simulink model "mc64_hb_43_newquant"  (Simulink 7.6)
settings: Solver=ode45  StartTime=0.0  StopTime=5000  RelTol=1e-3
libraries: xbsIndex_r4 x1281, xps_library x27, casper_library_misc x17, dspsigops x8
(part 2 of 13)

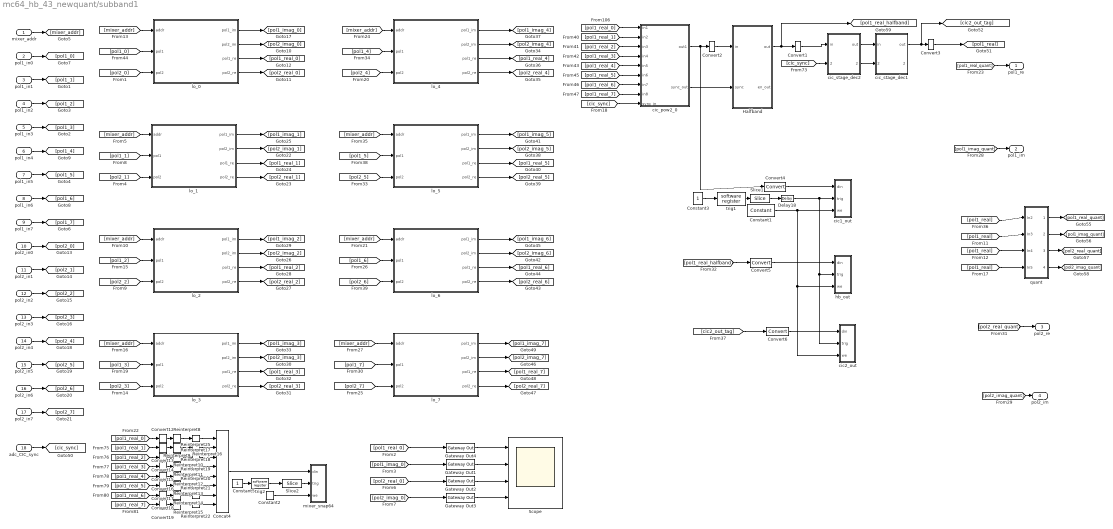
== system mc64_hb_43_newquant/subband1 ==
  mixer_addr : Inport
  pol1_in0 : Inport  Port=2
  pol1_in1 : Inport  Port=3
  pol1_in2 : Inport  Port=4
  pol1_in3 : Inport  Port=5
  pol1_in4 : Inport  Port=6
  pol1_in5 : Inport  Port=7
  pol1_in6 : Inport  Port=8
  pol1_in7 : Inport  Port=9
  pol2_in0 : Inport  Port=10
  pol2_in1 : Inport  Port=11
  pol2_in2 : Inport  Port=12
  pol2_in3 : Inport  Port=13
  pol2_in4 : Inport  Port=14
  pol2_in5 : Inport  Port=15
  pol2_in6 : Inport  Port=16
  pol2_in7 : Inport  Port=17
  adc_CIC_sync : Inport  Port=18
  Concat4 : xbsIndex_r4/Concat  num_inputs=8  dbl_ovrd=off  block_type=concat
  Constant1 : xbsIndex_r4/Constant  const=1  gui_display_data_type=Boolean  arith_type=Boolean  n_bits=16  bin_pt=14  preci_type=Single  exp_width=8  frac_width=24  explicit_period=off  period=1  equ=P=C  opselect=C  inp2=PCIN>>17  opr=+  inp1=P  carry=CIN  dbl_ovrd=off  block_type=constant
  Constant2 : xbsIndex_r4/Constant  const=1  gui_display_data_type=Boolean  arith_type=Boolean  n_bits=16  bin_pt=14  preci_type=Single  exp_width=8  frac_width=24  explicit_period=off  period=1  equ=P=C  opselect=C  inp2=PCIN>>17  opr=+  inp1=P  carry=CIN  dbl_ovrd=off  block_type=constant
  Constant3 : Constant
  Constant5 : Constant
  Convert1 : xbsIndex_r4/Convert  gui_display_data_type=Fixed-point  arith_type="Signed  (2's comp)"  n_bits=32  bin_pt=12  float_type=Single  exp_bits=8  fraction_bits=24  quantization=Truncate  overflow=Wrap  en=off  latency=1  dbl_ovrd=off  pipeline=off  block_type=convert
  Convert{12..19} (8 alike) : xbsIndex_r4/Convert  gui_display_data_type=Fixed-point  arith_type=Unsigned  n_bits=8  bin_pt=6  float_type=Single  exp_bits=8  fraction_bits=24  quantization=Truncate  overflow=Wrap  en=off  latency=2  dbl_ovrd=off  pipeline=off  block_type=convert
      settings: block_version=11.4
  Convert2 : xbsIndex_r4/Convert  gui_display_data_type=Fixed-point  arith_type="Signed  (2's comp)"  n_bits=32  bin_pt=18  float_type=Single  exp_bits=8  fraction_bits=24  quantization=Truncate  overflow=Wrap  en=off  latency=1  dbl_ovrd=off  pipeline=off  block_type=convert
  Convert3 : xbsIndex_r4/Convert  gui_display_data_type=Fixed-point  arith_type="Signed  (2's comp)"  n_bits=32  bin_pt=6  float_type=Single  exp_bits=8  fraction_bits=24  quantization=Truncate  overflow=Wrap  en=off  latency=1  dbl_ovrd=off  pipeline=off  block_type=convert
  Convert4 : xbsIndex_r4/Convert  gui_display_data_type=Fixed-point  arith_type="Signed  (2's comp)"  n_bits=64  bin_pt=22  float_type=Single  exp_bits=8  fraction_bits=24  quantization=Truncate  overflow=Wrap  en=off  latency=1  dbl_ovrd=off  pipeline=off  block_type=convert
  Convert5 : xbsIndex_r4/Convert  gui_display_data_type=Fixed-point  arith_type="Signed  (2's comp)"  n_bits=64  bin_pt=32  float_type=Single  exp_bits=8  fraction_bits=24  quantization=Truncate  overflow=Wrap  en=off  latency=1  dbl_ovrd=off  pipeline=off  block_type=convert
  Convert6 : xbsIndex_r4/Convert  gui_display_data_type=Fixed-point  arith_type="Signed  (2's comp)"  n_bits=64  bin_pt=12  float_type=Single  exp_bits=8  fraction_bits=24  quantization=Truncate  overflow=Wrap  en=off  latency=1  dbl_ovrd=off  pipeline=off  block_type=convert
  Delay18 : xbsIndex_r4/Delay  rst=off  infoeditControl=Selection of Reset will increase slice count due to use of real FFs and instead of SRLs  en=off  latency=20  dbl_ovrd=off  reg_retiming=off  block_type=delay
  Gateway Out{1..4} (4 alike) : xbsIndex_r4/Gateway Out  hdl_port=on  timing_constraint=None  locs_specified=off  LOCs={}  block_type=gatewayout
      settings: infoedit="Gateway out block.  Converts Xilinx fixed point or floating-point type inputs into ouputs of type Simulink integer, double, or fixed point.<br><br>Hardware notes:  In hardware these blocks become top level output ports or are discarded, depending on how they are configured."
  Halfband : Subsystem  AncestorBlock=gbt_library/Halfband  mask(Halfband FIR){mult_latency=3, add_latency=2, hold_period=2, passband=0.4, fir_len=17}
      mask prompts: mult_latency "Multiplication latency"; add_latency "Add latency"; hold_period "Hold Period"; passband "Width of Halfband passband (<0.5)"; fir_len "FIR Length (odd) [Number of Taps will be: 2*fir_len+1]"
      mask help: A halfband FIR for low rate computation.
      mask init:
      | coeffs = halfband_coeff_gen(fir_len, passband);
      | config.source=str2func('hold_fir_init_xblock');
      | config.depend=[get_dependlist('hold_fir'),{'halfband_coeff_gen'}];
      | config.toplevel=gcb;
      | set_param(gcb,'LinkStatus','inactive');
      | xBlock(config, {config.toplevel,...
      |     'mult_latency', mult_latency, ...
      |     'add_latency', add_latency, ...
      |     'hold_period', hold_period, ...
      |     'coeffs', coeffs});
      settings: AttributesFormatString=|
      | 35-tap FIR filter (19 nonzero tap)
      |  hold period: 2
      |  mult latency: 3
      |  add latency: 2
  Reinterpret{8..15} (8 alike) : xbsIndex_r4/Reinterpret  force_arith_type=on  arith_type="Signed  (2's comp)"  force_bin_pt=on  bin_pt=7  block_type=reinterpret
  Reinterpret{16..22,25} (8 alike) : xbsIndex_r4/Reinterpret  force_arith_type=on  arith_type=Unsigned  force_bin_pt=on  bin_pt=0  block_type=reinterpret
  Scope : Scope  NumInputPorts=4
      settings: YMin=-0.0075~-1~-0.0075~-1  YMax=0.0075~1~0.0075~1
  Slice1 : xbsIndex_r4/Slice  nbits=1  boolean_output=on  mode=Lower Bit Location + Width  bit1=0  base1=MSB of Input  bit0=0  base0=LSB of Input  dbl_ovrd=off  block_type=slice
  Slice2 : xbsIndex_r4/Slice  nbits=1  boolean_output=on  mode=Lower Bit Location + Width  bit1=0  base1=MSB of Input  bit0=0  base0=LSB of Input  dbl_ovrd=off  block_type=slice
  cic1_out : Subsystem  AncestorBlock=casper_library_scopes/snap64  mask(snap64){nsamples=13}
      mask prompts: nsamples "No. of samples(2^?)"
      mask help:
      | The <i>snap</i> block provides a packaged solution to capturing data from
      | the FPGA fabric and making it accessible from the CPU.  The block comes in
      | 2 flavors: <i>snap</i> (which captures to a 32 bit wide Shared BRAM), and
      | <i>snap64</i> (which captures to 2x32 bit wide Shared BRAMs to effect a
      | 64 bit capture).
      mask Help: eval('xlWeb(''http://casper.berkeley.edu/wiki/Snap'')')
  cic2_out : Subsystem  AncestorBlock=casper_library_scopes/snap64  mask(snap64){nsamples=13}
      mask prompts: nsamples "No. of samples(2^?)"
      mask help:
      | The <i>snap</i> block provides a packaged solution to capturing data from
      | the FPGA fabric and making it accessible from the CPU.  The block comes in
      | 2 flavors: <i>snap</i> (which captures to a 32 bit wide Shared BRAM), and
      | <i>snap64</i> (which captures to 2x32 bit wide Shared BRAMs to effect a
      | 64 bit capture).
      mask Help: eval('xlWeb(''http://casper.berkeley.edu/wiki/Snap'')')
  cic_pow2_0 : Subsystem  AncestorBlock=gbt_library/cic_pow2  mask(CIC (pow2)){n_stages=4, dec_rate=16, input_clk_period=1, n_inputs=8, add_latency=1, n_bits=8, bin_pt=7}
      mask prompts: n_stages "CIC filter Order"; dec_rate "Decimation rate"; input_clk_period "Input Clock Period"; n_inputs "Number of inputs"; add_latency "Add latency"; n_bits "Input bit width"; bin_pt "Binary point"
      mask help:
      | A non-recursive CIC filter with parallel inputs.
      | Supports decimation rate of power of 2.
      | A multi-stage implementation with each stage of decimation rate 2.
      mask init:
      | config.source = str2func('cic_pow2_init_xblock');
      | config.toplevel = gcb;
      | config.depend = get_dependlist('cic_pow2'); 
      | set_param(gcb,'LinkStatus','inactive');
      | xBlock(config, {config.toplevel,...
      |                 'n_stages',n_stages, ...
      |                 'dec_rate', dec_rate, ...
      |                 'input_clk_rate', input_clk_period, ...
      |                 'n_inputs', n_inputs,...
      |                 'add_latency',add_latency,...
      |                 'n_bits', n_bits, ...
      |                 'bin_pt', bin_pt} ...
      |                 );
      | disp('new block added');
      settings: AttributesFormatString=|
      | dec_rate = 16
      | Order = 4
  cic_stage_dec1 : Subsystem  AncestorBlock=gbt_library/cic_stage_dec2  mask(CIC stage (dec2)){n_stages=3, recursive=off, dec_rate=2, n_inputs=1, input_clk_period=1, input_period=4, add_latency=2, n_bits=8, bin_pt=7}
      mask prompts: n_stages "CIC filter Order"; recursive "Recursive?"; dec_rate "Decimation rate"; n_inputs "Number of Inputs"; input_clk_period "Input Clock period (Actual)"; input_period "Effective Input Sampling Period"; add_latency "Add latency"; n_bits "Input bit width"; bin_pt "Binary point"
      mask help:
      | A single stage of CIC filter with even number of parallel inputs.
      | Only supports decimation rate = 2.
      | If n_inputs > 1, number of outputs = n_inputs/2.
      | Non-recursive.
      |
      | Clock period:
      | input_clk_period is the actual sampling period of incoming data stream.
      | input_period is the effective (or expected) sampling period of incoming data stream.
      | E.g. For incoming data stream X[n] = [1& 1 2 2 3 3 4 4 5 5 ...], the input_clk_period is 1 and the input_period is 2.
      mask init:
      | if recursive
      |     % recursive case
      |     config.source=str2func('cic_stage_dec2_recursive_init_xblock');
      |     config.toplevel=gcb;
      |     config.depend = get_dependlist('cic_stage_dec2_recursive');
      |     set_param(gcb,'LinkStatus','inactive');
      |     xBlock(config, {config.toplevel, ...
      |                 'n_stages', n_stages, ...
      |                 'dec_rate', dec_rate, ...
      |                 'n_inputs', n_inputs, ...
      |                 'input_clk_period', input_clk_period, ...
      |                 'input_period', input_period, ...
      |                 'add_latency', add_latency, ...
      |                 'input_bits', n_bits, ...
      |                 'bin_pt', bin_pt, ...
      |                 'delay_len', 1});
      | else
      |     % non-recursive case
      |     config.source=str2func('cic_stage_dec2_init_xblock');
      |     config.toplevel=gcb;
      |     config.depend = get_dependlist('cic_stage_dec2');
      |     set_param(gcb,'LinkStatus','inactive');
      |     xBlock(config, {config.toplevel, ...
      |                 'n_stages', n_stages, ...
      |                 'dec_rate', dec_rate, ...
      |                 'n_inputs', n_inputs, ...
      |                 'input_clk_period', input_clk_period, ...
      |                 'input_period', input_period, ...
      |                 'add_latency', add_latency, ...
      |                 'n_bits', n_bits, ...
      |                 'bin_pt', bin_pt});
      | end
      settings: AttributesFormatString=|
      | nonrecursive
      | 8_7_in
      | clock(actualy/effective): 1/4
      mask CallbackString:
      | ||n=get_param(gcb,'dec_rate');
      | if ~isempty(n)
      |     n = eval(n);
      |     if ~isprime(n) && n~=1
      |         errordlg('Only supports decimation rate that is a prime number or 1');
      |         set_param(gcb,'dec_rate','');
      |     end
      | end||||||
  cic_stage_dec2 : Subsystem  AncestorBlock=gbt_library/cic_stage_dec2  mask(CIC stage (dec2)){n_stages=3, recursive=off, dec_rate=2, n_inputs=1, input_clk_period=1, input_period=2, add_latency=2, n_bits=8, bin_pt=7}
      mask prompts: n_stages "CIC filter Order"; recursive "Recursive?"; dec_rate "Decimation rate"; n_inputs "Number of Inputs"; input_clk_period "Input Clock period (Actual)"; input_period "Effective Input Sampling Period"; add_latency "Add latency"; n_bits "Input bit width"; bin_pt "Binary point"
      mask help:
      | A single stage of CIC filter with even number of parallel inputs.
      | Only supports decimation rate = 2.
      | If n_inputs > 1, number of outputs = n_inputs/2.
      | Non-recursive.
      |
      | Clock period:
      | input_clk_period is the actual sampling period of incoming data stream.
      | input_period is the effective (or expected) sampling period of incoming data stream.
      | E.g. For incoming data stream X[n] = [1& 1 2 2 3 3 4 4 5 5 ...], the input_clk_period is 1 and the input_period is 2.
      mask init: same as mc64_hb_43_newquant/subband1/cic_stage_dec1
      settings: AttributesFormatString=|
      | nonrecursive
      | 8_7_in
      | clock(actualy/effective): 1/2
      mask CallbackString:
      | ||n=get_param(gcb,'dec_rate');
      | if ~isempty(n)
      |     n = eval(n);
      |     if ~isprime(n) && n~=1
      |         errordlg('Only supports decimation rate that is a prime number or 1');
      |         set_param(gcb,'dec_rate','');
      |     end
      | end||||||
  hb_out : Subsystem  AncestorBlock=casper_library_scopes/snap64  mask(snap64){nsamples=13}
      mask prompts: nsamples "No. of samples(2^?)"
      mask help:
      | The <i>snap</i> block provides a packaged solution to capturing data from
      | the FPGA fabric and making it accessible from the CPU.  The block comes in
      | 2 flavors: <i>snap</i> (which captures to a 32 bit wide Shared BRAM), and
      | <i>snap64</i> (which captures to 2x32 bit wide Shared BRAMs to effect a
      | 64 bit capture).
      mask Help: eval('xlWeb(''http://casper.berkeley.edu/wiki/Snap'')')
  lo_0 : Subsystem  AncestorBlock=gbt_library/complex_mix_lo
  lo_1 : Subsystem  AncestorBlock=gbt_library/complex_mix_lo
  lo_2 : Subsystem  AncestorBlock=gbt_library/complex_mix_lo
  lo_3 : Subsystem  AncestorBlock=gbt_library/complex_mix_lo
  lo_4 : Subsystem  AncestorBlock=gbt_library/complex_mix_lo
  lo_5 : Subsystem  AncestorBlock=gbt_library/complex_mix_lo
  lo_6 : Subsystem  AncestorBlock=gbt_library/complex_mix_lo
  lo_7 : Subsystem  AncestorBlock=gbt_library/complex_mix_lo
  mixer_snap64 : Subsystem  AncestorBlock=casper_library_scopes/snap64  mask(snap64){nsamples=11}
      mask prompts: nsamples "No. of samples(2^?)"
      mask help:
      | The <i>snap</i> block provides a packaged solution to capturing data from
      | the FPGA fabric and making it accessible from the CPU.  The block comes in
      | 2 flavors: <i>snap</i> (which captures to a 32 bit wide Shared BRAM), and
      | <i>snap64</i> (which captures to 2x32 bit wide Shared BRAMs to effect a
      | 64 bit capture).
      mask Help: eval('xlWeb(''http://casper.berkeley.edu/wiki/Snap'')')
  quant : Subsystem
  trig1 : xps_library/software register  Tag=xps:sw_reg  SystemSampleTime=-1  io_dir=From Processor  arith_type=Unsigned  bitwidth=32  bin_pt=0  sample_period=1  gw_name=mc64_hb_43_noise_subband1_trig1_user_data_out
      link override cic_filter_testing_to_compile_trig_user_data_out: arith_type=Unsigned  n_bits=32  bin_pt=0  period=1
  trig2 : xps_library/software register  Tag=xps:sw_reg  SystemSampleTime=-1  io_dir=From Processor  arith_type=Unsigned  bitwidth=32  bin_pt=0  sample_period=1  gw_name=mc64_hb_43_noise_subband1_trig2_user_data_out
      link override cic_filter_testing_to_compile_trig_user_data_out: arith_type=Unsigned  n_bits=32  bin_pt=0  period=1
  pol1_re : Outport
  pol1_im : Outport  Port=2
  pol2_re : Outport  Port=3
  pol2_im : Outport  Port=4
  wires:
  mixer_addr/1 -> [mixer_addr]
  pol1_in0/1 -> [pol1_0]
  [pol1_real_0] -> cic_pow2_0/1(in1)
  pol1_in1/1 -> [pol1_1]
  pol1_in2/1 -> [pol1_2]
  pol1_in3/1 -> [pol1_3]
  pol1_in4/1 -> [pol1_4]
  pol1_in5/1 -> [pol1_5]
  pol1_in6/1 -> [pol1_6]
  pol1_in7/1 -> [pol1_7]
  pol2_in0/1 -> [pol2_0]
  pol2_in1/1 -> [pol2_1]
  pol2_in2/1 -> [pol2_2]
  pol2_in3/1 -> [pol2_3]
  pol2_in4/1 -> [pol2_4]
  pol2_in5/1 -> [pol2_5]
  pol2_in6/1 -> [pol2_6]
  pol2_in7/1 -> [pol2_7]
  [mixer_addr] -> lo_1/1(addr)
  [mixer_addr] -> lo_2/1(addr)
  [mixer_addr] -> lo_3/1(addr)
  [pol1_real_1] -> cic_pow2_0/2(in2)
  [pol1_real_2] -> cic_pow2_0/3(in3)
  [pol1_real_3] -> cic_pow2_0/4(in4)
  [pol1_real_4] -> cic_pow2_0/5(in5)
  [pol1_real_5] -> cic_pow2_0/6(in6)
  [pol1_real_6] -> cic_pow2_0/7(in7)
  [pol1_real_7] -> cic_pow2_0/8(in8)
  lo_4/1(pol1_im) -> [pol1_imag_4]
  lo_4/2(pol2_im) -> [pol2_imag_4]
  lo_4/3(pol1_re) -> [pol1_real_4]
  lo_4/4(pol2_re) -> [pol2_real_4]
  [mixer_addr] -> lo_4/1(addr)
  [pol2_4] -> lo_4/3(pol2)
  [pol1_4] -> lo_4/2(pol1)
  [mixer_addr] -> lo_0/1(addr)
  [pol1_0] -> lo_0/2(pol1)
  [pol2_0] -> lo_0/3(pol2)
  lo_0/1(pol1_im) -> [pol1_imag_0]
  lo_0/2(pol2_im) -> [pol2_imag_0]
  lo_0/3(pol1_re) -> [pol1_real_0]
  lo_0/4(pol2_re) -> [pol2_real_0]
  [pol1_1] -> lo_1/2(pol1)
  [pol2_1] -> lo_1/3(pol2)
  lo_1/1(pol1_im) -> [pol1_imag_1]
  lo_1/2(pol2_im) -> [pol2_imag_1]
  lo_1/3(pol1_re) -> [pol1_real_1]
  lo_1/4(pol2_re) -> [pol2_real_1]
  [pol1_2] -> lo_2/2(pol1)
  [pol2_2] -> lo_2/3(pol2)
  [pol1_3] -> lo_3/2(pol1)
  [pol2_3] -> lo_3/3(pol2)
  lo_3/1(pol1_im) -> [pol1_imag_3]
  lo_3/2(pol2_im) -> [pol2_imag_3]
  lo_3/3(pol1_re) -> [pol1_real_3]
  lo_3/4(pol2_re) -> [pol2_real_3]
  [mixer_addr] -> lo_5/1(addr)
  [pol1_5] -> lo_5/2(pol1)
  [pol2_5] -> lo_5/3(pol2)
  lo_5/1(pol1_im) -> [pol1_imag_5]
  lo_5/2(pol2_im) -> [pol2_imag_5]
  lo_5/3(pol1_re) -> [pol1_real_5]
  lo_5/4(pol2_re) -> [pol2_real_5]
  [mixer_addr] -> lo_6/1(addr)
  [pol1_6] -> lo_6/2(pol1)
  [pol2_6] -> lo_6/3(pol2)
  lo_6/1(pol1_im) -> [pol1_imag_6]
  lo_6/2(pol2_im) -> [pol2_imag_6]
  lo_6/3(pol1_re) -> [pol1_real_6]
  lo_6/4(pol2_re) -> [pol2_real_6]
  [mixer_addr] -> lo_7/1(addr)
  [pol1_7] -> lo_7/2(pol1)
  [pol2_7] -> lo_7/3(pol2)
  lo_7/1(pol1_im) -> [pol1_imag_7]
  lo_7/2(pol2_im) -> [pol2_imag_7]
  lo_7/3(pol1_re) -> [pol1_real_7]
  lo_7/4(pol2_re) -> [pol2_real_7]
  lo_2/1(pol1_im) -> [pol1_imag_2]
  lo_2/2(pol2_im) -> [pol2_imag_2]
  lo_2/3(pol1_re) -> [pol1_real_2]
  lo_2/4(pol2_re) -> [pol2_real_2]
  [pol1_real_0] -> Gateway Out4/1
  [pol1_imag_0] -> Gateway Out1/1
  [pol2_real_0] -> Gateway Out2/1
  [pol2_imag_0] -> Gateway Out3/1
  Gateway Out4/1 -> Scope/1
  Gateway Out1/1 -> Scope/2
  Gateway Out2/1 -> Scope/3
  Gateway Out3/1 -> Scope/4
  adc_CIC_sync/1 -> [cic_sync]
  [cic_sync] -> cic_pow2_0/9(sync_in)
  Concat4/1 -> mixer_snap64/1(din)
  Constant2/1 -> mixer_snap64/3(we)
  Convert12/1 -> Reinterpret8/1
  [pol1_real_0] -> Convert12/1
  Reinterpret8/1 -> Reinterpret25/1
  Convert13/1 -> Reinterpret9/1
  [pol1_real_1] -> Convert13/1
  Reinterpret9/1 -> Reinterpret16/1
  Convert14/1 -> Reinterpret10/1
  [pol1_real_2] -> Convert14/1
  Reinterpret10/1 -> Reinterpret17/1
  Convert15/1 -> Reinterpret11/1
  [pol1_real_3] -> Convert15/1
  Reinterpret11/1 -> Reinterpret18/1
  Convert16/1 -> Reinterpret12/1
  [pol1_real_4] -> Convert16/1
  Reinterpret12/1 -> Reinterpret19/1
  Convert17/1 -> Reinterpret13/1
  [pol1_real_5] -> Convert17/1
  Reinterpret13/1 -> Reinterpret20/1
  Convert18/1 -> Reinterpret14/1
  [pol1_real_6] -> Convert18/1
  Reinterpret14/1 -> Reinterpret21/1
  Convert19/1 -> Reinterpret15/1
  [pol1_real_7] -> Convert19/1
  Reinterpret15/1 -> Reinterpret22/1
  Reinterpret25/1 -> Concat4/1
  Reinterpret16/1 -> Concat4/2
  Reinterpret17/1 -> Concat4/3
  Reinterpret18/1 -> Concat4/4
  Reinterpret19/1 -> Concat4/5
  Reinterpret20/1 -> Concat4/6
  Reinterpret21/1 -> Concat4/7
  Reinterpret22/1 -> Concat4/8
  Constant5/1 -> trig2/1
  trig2/1 -> Slice2/1
  Slice2/1 -> mixer_snap64/2(trig)
  [pol1_real_quant] -> pol1_re/1
  cic_pow2_0/2(sync_out) -> Halfband/2(sync)
  cic_stage_dec2/2(sync_out) -> cic_stage_dec1/2(sync_in)
  cic_stage_dec2/1(out) -> cic_stage_dec1/1(in)
  Halfband/1(out) -> Convert1/1, [pol1_real_halfband]
  cic_stage_dec1/1(out) -> Convert3/1, [cic2_out_tag]
  [cic_sync] -> cic_stage_dec2/2(sync_in)
  cic_pow2_0/1(out1) -> Convert2/1, Convert4/1
  Convert2/1 -> Halfband/1(in)
  Convert1/1 -> cic_stage_dec2/1(in)
  Convert3/1 -> [pol1_real]
  [pol1_imag_quant] -> pol1_im/1
  quant/1(Out1) -> [pol1_real_quant]
  quant/2(Out2) -> [pol1_imag_quant]
  [pol1_real] -> quant/1(In2)
  [pol1_real] -> quant/2(In3)
  [pol1_real] -> quant/3(In4)
  [pol1_real] -> quant/4(In5)
  quant/3(Out3) -> [pol2_real_quant]
  quant/4(Out4) -> [pol2_imag_quant]
  [pol2_real_quant] -> pol2_re/1
  [pol2_imag_quant] -> pol2_im/1
  Constant1/1 -> cic1_out/3(we), hb_out/3(we), cic2_out/3(we)
  Constant3/1 -> trig1/1
  trig1/1 -> Slice1/1
  Slice1/1 -> Delay18/1
  Delay18/1 -> cic1_out/2(trig), hb_out/2(trig), cic2_out/2(trig)
  Convert4/1 -> cic1_out/1(din)
  [pol1_real_halfband] -> Convert5/1
  Convert5/1 -> hb_out/1(din)
  [cic2_out_tag] -> Convert6/1
  Convert6/1 -> cic2_out/1(din)

== system mc64_hb_43_newquant/adc083000x2/adc0_sim ==
  sim_adc_data_in : Inport
  adc_bias : Bias  Bias=128  SaturateOnIntegerOverflow=on
  adc_gain : Gain  Gain=128
  overflow_detector : Subsystem  AncestorBlock=casper_library/Misc/of_detect_bus  mask(of_detect_bus){nStreams=8, bit_width=8}
      mask prompts: nStreams "Number of Streams"; bit_width "Bit Width"
      mask init:
      | adc_overflow_detector_init(gcb, ...
      |     'nStreams', nStreams, ...
      |     'bit_width', bit_width);
  sample0_ds : dspsigops/Downsample  N=8  phase=1  InputProcessing=Inherited (this choice will be removed - see release notes)  RateOptions=Enforce single-rate processing  smode=Force single rate  fmode=Maintain input frame size  ic=0
  sample1_ds : dspsigops/Downsample  N=8  phase=2  InputProcessing=Inherited (this choice will be removed - see release notes)  RateOptions=Enforce single-rate processing  smode=Force single rate  fmode=Maintain input frame size  ic=0
  sample2_ds : dspsigops/Downsample  N=8  phase=3  InputProcessing=Inherited (this choice will be removed - see release notes)  RateOptions=Enforce single-rate processing  smode=Force single rate  fmode=Maintain input frame size  ic=0
  sample3_ds : dspsigops/Downsample  N=8  phase=4  InputProcessing=Inherited (this choice will be removed - see release notes)  RateOptions=Enforce single-rate processing  smode=Force single rate  fmode=Maintain input frame size  ic=0
  sample4_ds : dspsigops/Downsample  N=8  phase=5  InputProcessing=Inherited (this choice will be removed - see release notes)  RateOptions=Enforce single-rate processing  smode=Force single rate  fmode=Maintain input frame size  ic=0
  sample5_ds : dspsigops/Downsample  N=8  phase=6  InputProcessing=Inherited (this choice will be removed - see release notes)  RateOptions=Enforce single-rate processing  smode=Force single rate  fmode=Maintain input frame size  ic=0
  sample6_ds : dspsigops/Downsample  N=8  phase=7  InputProcessing=Inherited (this choice will be removed - see release notes)  RateOptions=Enforce single-rate processing  smode=Force single rate  fmode=Maintain input frame size  ic=0
  sample7_ds : dspsigops/Downsample  N=8  phase=0  InputProcessing=Inherited (this choice will be removed - see release notes)  RateOptions=Enforce single-rate processing  smode=Force single rate  fmode=Maintain input frame size  ic=0
  s0 : Outport
  s1 : Outport  Port=2
  s2 : Outport  Port=3
  s3 : Outport  Port=4
  s4 : Outport  Port=5
  s5 : Outport  Port=6
  s6 : Outport  Port=7
  s7 : Outport  Port=8
  of : Outport  Port=9
  wires:
  sim_adc_data_in/1 -> adc_gain/1
  adc_gain/1 -> adc_bias/1
  overflow_detector/1(overflow) -> of/1
  adc_bias/1 -> sample0_ds/1, sample1_ds/1, sample2_ds/1, sample3_ds/1, sample4_ds/1, sample5_ds/1, sample6_ds/1, sample7_ds/1
  sample0_ds/1 -> overflow_detector/1(s0), s0/1
  sample1_ds/1 -> overflow_detector/2(s1), s1/1
  sample2_ds/1 -> overflow_detector/3(s2), s2/1
  sample3_ds/1 -> overflow_detector/4(s3), s3/1
  sample4_ds/1 -> overflow_detector/5(s4), s4/1
  sample5_ds/1 -> overflow_detector/6(s5), s5/1
  sample6_ds/1 -> overflow_detector/7(s6), s6/1
  sample7_ds/1 -> overflow_detector/8(s7), s7/1

== system mc64_hb_43_newquant/adc_snap64/bram_lsb ==
  addr : Inport
  data_in : Inport  Port=2
  we : Inport  Port=3
  calc_add : Subsystem
  convert_addr : xbsIndex_r4/Convert  gui_display_data_type=Fixed-point  arith_type=Unsigned  n_bits=addr_width  bin_pt=0  float_type=Single  exp_bits=8  fraction_bits=24  quantization=Truncate  overflow=Wrap  en=off  latency=0  dbl_ovrd=off  pipeline=off  block_type=convert
      settings: xl_area=[0, 0, 0, 0, 0, 0, 0]
  convert_din : xbsIndex_r4/Convert  gui_display_data_type=Fixed-point  arith_type=Unsigned  n_bits=data_width  bin_pt=data_bin_pt  float_type=Single  exp_bits=8  fraction_bits=24  quantization=Truncate  overflow=Wrap  en=off  latency=0  dbl_ovrd=off  pipeline=off  block_type=convert
      settings: xl_area=[0, 0, 0, 0, 0, 0, 0]
  convert_din1 : xbsIndex_r4/Convert  gui_display_data_type=Fixed-point  arith_type=Unsigned  n_bits=data_width  bin_pt=data_bin_pt  float_type=Single  exp_bits=8  fraction_bits=24  quantization=Truncate  overflow=Wrap  en=off  latency=0  dbl_ovrd=off  pipeline=off  block_type=convert
      settings: xl_area=[0, 0, 0, 0, 0, 0, 0]
  convert_we : xbsIndex_r4/Convert  gui_display_data_type=Fixed-point  arith_type=Unsigned  n_bits=1  bin_pt=0  float_type=Single  exp_bits=8  fraction_bits=24  quantization=Truncate  overflow=Wrap  en=off  latency=0  dbl_ovrd=off  pipeline=off  block_type=convert
      settings: xl_area=[0, 0, 0, 0, 0, 0, 0]
  mc64_hb_43_noise_adc_snap64_bram_lsb_addr : xbsIndex_r4/Gateway Out  hdl_port=on  timing_constraint=None  locs_specified=off  LOCs={'A5','B9','A9','C1','A3','G6','E9','A6','A7','A8','B8','B1','B3','D9','B5','B4','B6','C2'}  block_type=gatewayout
      settings: infoedit="Gateway out block.  Converts Xilinx fixed point inputs into ouputs of type Simulink integer, double, or fixed point.<P><P>Hardware notes:  In hardware these blocks become top level output ports or are discarded, depending on how they are configured."  xl_area=[0, 0, 0, 0, 0, 0, 0]  sginterface={'Nallatech'=>{'xdspkit'=>{'non_memory_mapped_port'=>'uprev_Shared_BRAM_addr'}},'Xilinx'=>{'jtaghwcosim'=>{'non_memory_mapped_port'=>'uprev_Shared_BRAM_addr'},'xdspkit'=>{'non_memory_mapped_port'=>'uprev_Shared_BRAM_addr'}}}
  mc64_hb_43_noise_adc_snap64_bram_lsb_data_in : xbsIndex_r4/Gateway Out  hdl_port=on  timing_constraint=None  locs_specified=off  LOCs={'B21','B22','A22','B23','B19','C19','A20','A21','A23','B24','A24','A25','E18','D18','C18','B18'}  block_type=gatewayout
      settings: infoedit="Gateway out block.  Converts Xilinx fixed point inputs into ouputs of type Simulink integer, double, or fixed point.<P><P>Hardware notes:  In hardware these blocks become top level output ports or are discarded, depending on how they are configured."  xl_area=[0, 0, 0, 0, 0, 0, 0]  sginterface={'Nallatech'=>{'xdspkit'=>{'non_memory_mapped_port'=>'uprev_Shared_BRAM_data_in'}},'Xilinx'=>{'jtaghwcosim'=>{'non_memory_mapped_port'=>'uprev_Shared_BRAM_data_in'},'xdspkit'=>{'non_memory_mapped_port'=>'uprev_Shared_BRAM_data_in'}}}
  mc64_hb_43_noise_adc_snap64_bram_lsb_data_out : xbsIndex_r4/Gateway In  gui_display_data_type=Fixed-point  arith_type=Unsigned  n_bits=data_width  bin_pt=data_bin_pt  preci_type=Single  exp_width=8  frac_width=24  quantization=Truncate  overflow=Wrap  period=sample_rate  dbl_ovrd=off  timing_constraint=None  locs_specified=off  LOCs={}  hdl_port=on  block_type=gatewayin
      settings: infoedit="Gateway in block.  Converts inputs of type Simulink integer, double and fixed point to  Xilinx fixed point type.<br><br>Hardware notes:  In hardware these blocks become top level input ports."  xl_area=[0, 0, 0, 0, 0, 0, 0]
  mc64_hb_43_noise_adc_snap64_bram_lsb_we : xbsIndex_r4/Gateway Out  hdl_port=on  timing_constraint=None  locs_specified=off  LOCs={'A14'}  block_type=gatewayout
      settings: infoedit="Gateway out block.  Converts Xilinx fixed point inputs into ouputs of type Simulink integer, double, or fixed point.<P><P>Hardware notes:  In hardware these blocks become top level output ports or are discarded, depending on how they are configured."  xl_area=[0, 0, 0, 0, 0, 0, 0]
  mem : Subsystem
  munge_in : Subsystem  AncestorBlock=casper_library_flow_control/munge  mask(munge){divisions=1, div_size=32, order=[0]}
      mask prompts: divisions "Number of divisions"; div_size "Division size (bits)"; order "Division packing order"
      mask help: Splits an input bus into the specified number of divisions and then recombines them in the order specified (most significant division = 0,least = number divisions-1)
      mask init:
      | munge_init(gcb, ...
      |     'divisions', divisions, ...
      |     'div_size', div_size, ...
      |     'order', order);
      settings: AttributesFormatString=|
      | [0]
      | 32 bits
  munge_out : Subsystem  AncestorBlock=casper_library_flow_control/munge  mask(munge){divisions=1, div_size=32, order=[0]}
      mask prompts: divisions "Number of divisions"; div_size "Division size (bits)"; order "Division packing order"
      mask help: Splits an input bus into the specified number of divisions and then recombines them in the order specified (most significant division = 0,least = number divisions-1)
      mask init:
      | munge_init(gcb, ...
      |     'divisions', divisions, ...
      |     'div_size', div_size, ...
      |     'order', order);
      settings: AttributesFormatString=|
      | [0]
      | 32 bits
  data_out : Outport
  wires:
  convert_din/1 -> munge_in/1(din)
  convert_din1/1 -> mc64_hb_43_noise_adc_snap64_bram_lsb_data_in/1
  convert_addr/1 -> mc64_hb_43_noise_adc_snap64_bram_lsb_addr/1
  calc_add/1(out) -> convert_addr/1
  munge_out/1(dout) -> data_out/1
  munge_in/1(dout) -> convert_din1/1
  mc64_hb_43_noise_adc_snap64_bram_lsb_we/1 -> mem/3(In3)
  mc64_hb_43_noise_adc_snap64_bram_lsb_data_in/1 -> mem/2(In2)
  mc64_hb_43_noise_adc_snap64_bram_lsb_addr/1 -> mem/1(In1)
  convert_we/1 -> mc64_hb_43_noise_adc_snap64_bram_lsb_we/1
  we/1 -> convert_we/1
  addr/1 -> calc_add/1(in)
  mc64_hb_43_noise_adc_snap64_bram_lsb_data_out/1 -> munge_out/1(din)
  data_in/1 -> convert_din/1
  mem/1(Out1) -> mc64_hb_43_noise_adc_snap64_bram_lsb_data_out/1

== system mc64_hb_43_newquant/adc_snap64/bram_msb ==
  addr : Inport
  data_in : Inport  Port=2
  we : Inport  Port=3
  calc_add : Subsystem
  convert_addr : xbsIndex_r4/Convert  gui_display_data_type=Fixed-point  arith_type=Unsigned  n_bits=addr_width  bin_pt=0  float_type=Single  exp_bits=8  fraction_bits=24  quantization=Truncate  overflow=Wrap  en=off  latency=0  dbl_ovrd=off  pipeline=off  block_type=convert
      settings: xl_area=[0, 0, 0, 0, 0, 0, 0]
  convert_din : xbsIndex_r4/Convert  gui_display_data_type=Fixed-point  arith_type=Unsigned  n_bits=data_width  bin_pt=data_bin_pt  float_type=Single  exp_bits=8  fraction_bits=24  quantization=Truncate  overflow=Wrap  en=off  latency=0  dbl_ovrd=off  pipeline=off  block_type=convert
      settings: xl_area=[0, 0, 0, 0, 0, 0, 0]
  convert_din1 : xbsIndex_r4/Convert  gui_display_data_type=Fixed-point  arith_type=Unsigned  n_bits=data_width  bin_pt=data_bin_pt  float_type=Single  exp_bits=8  fraction_bits=24  quantization=Truncate  overflow=Wrap  en=off  latency=0  dbl_ovrd=off  pipeline=off  block_type=convert
      settings: xl_area=[0, 0, 0, 0, 0, 0, 0]
  convert_we : xbsIndex_r4/Convert  gui_display_data_type=Fixed-point  arith_type=Unsigned  n_bits=1  bin_pt=0  float_type=Single  exp_bits=8  fraction_bits=24  quantization=Truncate  overflow=Wrap  en=off  latency=0  dbl_ovrd=off  pipeline=off  block_type=convert
      settings: xl_area=[0, 0, 0, 0, 0, 0, 0]
  mc64_hb_43_noise_adc_snap64_bram_msb_addr : xbsIndex_r4/Gateway Out  hdl_port=on  timing_constraint=None  locs_specified=off  LOCs={'A5','B9','A9','C1','A3','G6','E9','A6','A7','A8','B8','B1','B3','D9','B5','B4','B6','C2'}  block_type=gatewayout
      settings: infoedit="Gateway out block.  Converts Xilinx fixed point inputs into ouputs of type Simulink integer, double, or fixed point.<P><P>Hardware notes:  In hardware these blocks become top level output ports or are discarded, depending on how they are configured."  xl_area=[0, 0, 0, 0, 0, 0, 0]  sginterface={'Nallatech'=>{'xdspkit'=>{'non_memory_mapped_port'=>'uprev_Shared_BRAM_addr'}},'Xilinx'=>{'jtaghwcosim'=>{'non_memory_mapped_port'=>'uprev_Shared_BRAM_addr'},'xdspkit'=>{'non_memory_mapped_port'=>'uprev_Shared_BRAM_addr'}}}
  mc64_hb_43_noise_adc_snap64_bram_msb_data_in : xbsIndex_r4/Gateway Out  hdl_port=on  timing_constraint=None  locs_specified=off  LOCs={'B21','B22','A22','B23','B19','C19','A20','A21','A23','B24','A24','A25','E18','D18','C18','B18'}  block_type=gatewayout
      settings: infoedit="Gateway out block.  Converts Xilinx fixed point inputs into ouputs of type Simulink integer, double, or fixed point.<P><P>Hardware notes:  In hardware these blocks become top level output ports or are discarded, depending on how they are configured."  xl_area=[0, 0, 0, 0, 0, 0, 0]  sginterface={'Nallatech'=>{'xdspkit'=>{'non_memory_mapped_port'=>'uprev_Shared_BRAM_data_in'}},'Xilinx'=>{'jtaghwcosim'=>{'non_memory_mapped_port'=>'uprev_Shared_BRAM_data_in'},'xdspkit'=>{'non_memory_mapped_port'=>'uprev_Shared_BRAM_data_in'}}}
  mc64_hb_43_noise_adc_snap64_bram_msb_data_out : xbsIndex_r4/Gateway In  gui_display_data_type=Fixed-point  arith_type=Unsigned  n_bits=data_width  bin_pt=data_bin_pt  preci_type=Single  exp_width=8  frac_width=24  quantization=Truncate  overflow=Wrap  period=sample_rate  dbl_ovrd=off  timing_constraint=None  locs_specified=off  LOCs={}  hdl_port=on  block_type=gatewayin
      settings: infoedit="Gateway in block.  Converts inputs of type Simulink integer, double and fixed point to  Xilinx fixed point type.<br><br>Hardware notes:  In hardware these blocks become top level input ports."  xl_area=[0, 0, 0, 0, 0, 0, 0]
  mc64_hb_43_noise_adc_snap64_bram_msb_we : xbsIndex_r4/Gateway Out  hdl_port=on  timing_constraint=None  locs_specified=off  LOCs={'A14'}  block_type=gatewayout
      settings: infoedit="Gateway out block.  Converts Xilinx fixed point inputs into ouputs of type Simulink integer, double, or fixed point.<P><P>Hardware notes:  In hardware these blocks become top level output ports or are discarded, depending on how they are configured."  xl_area=[0, 0, 0, 0, 0, 0, 0]
  mem : Subsystem
  munge_in : Subsystem  AncestorBlock=casper_library_flow_control/munge  mask(munge){divisions=1, div_size=32, order=[0]}
      mask prompts: divisions "Number of divisions"; div_size "Division size (bits)"; order "Division packing order"
      mask help: Splits an input bus into the specified number of divisions and then recombines them in the order specified (most significant division = 0,least = number divisions-1)
      mask init:
      | munge_init(gcb, ...
      |     'divisions', divisions, ...
      |     'div_size', div_size, ...
      |     'order', order);
      settings: AttributesFormatString=|
      | [0]
      | 32 bits
  munge_out : Subsystem  AncestorBlock=casper_library_flow_control/munge  mask(munge){divisions=1, div_size=32, order=[0]}
      mask prompts: divisions "Number of divisions"; div_size "Division size (bits)"; order "Division packing order"
      mask help: Splits an input bus into the specified number of divisions and then recombines them in the order specified (most significant division = 0,least = number divisions-1)
      mask init:
      | munge_init(gcb, ...
      |     'divisions', divisions, ...
      |     'div_size', div_size, ...
      |     'order', order);
      settings: AttributesFormatString=|
      | [0]
      | 32 bits
  data_out : Outport
  wires:
  convert_din/1 -> munge_in/1(din)
  convert_din1/1 -> mc64_hb_43_noise_adc_snap64_bram_msb_data_in/1
  convert_addr/1 -> mc64_hb_43_noise_adc_snap64_bram_msb_addr/1
  calc_add/1(out) -> convert_addr/1
  munge_out/1(dout) -> data_out/1
  munge_in/1(dout) -> convert_din1/1
  mc64_hb_43_noise_adc_snap64_bram_msb_we/1 -> mem/3(In3)
  mc64_hb_43_noise_adc_snap64_bram_msb_data_in/1 -> mem/2(In2)
  mc64_hb_43_noise_adc_snap64_bram_msb_addr/1 -> mem/1(In1)
  convert_we/1 -> mc64_hb_43_noise_adc_snap64_bram_msb_we/1
  we/1 -> convert_we/1
  addr/1 -> calc_add/1(in)
  mc64_hb_43_noise_adc_snap64_bram_msb_data_out/1 -> munge_out/1(din)
  data_in/1 -> convert_din/1
  mem/1(Out1) -> mc64_hb_43_noise_adc_snap64_bram_msb_data_out/1

== system mc64_hb_43_newquant/snap1/bram ==
  addr : Inport
  data_in : Inport  Port=2
  we : Inport  Port=3
  calc_add : Subsystem
  convert_addr : xbsIndex_r4/Convert  gui_display_data_type=Fixed-point  arith_type=Unsigned  n_bits=addr_width  bin_pt=0  float_type=Single  exp_bits=8  fraction_bits=24  quantization=Truncate  overflow=Wrap  en=off  latency=0  dbl_ovrd=off  pipeline=off  block_type=convert
      settings: xl_area=[0, 0, 0, 0, 0, 0, 0]
  convert_din : xbsIndex_r4/Convert  gui_display_data_type=Fixed-point  arith_type=Unsigned  n_bits=data_width  bin_pt=data_bin_pt  float_type=Single  exp_bits=8  fraction_bits=24  quantization=Truncate  overflow=Wrap  en=off  latency=0  dbl_ovrd=off  pipeline=off  block_type=convert
      settings: xl_area=[0, 0, 0, 0, 0, 0, 0]
  convert_din1 : xbsIndex_r4/Convert  gui_display_data_type=Fixed-point  arith_type=Unsigned  n_bits=data_width  bin_pt=data_bin_pt  float_type=Single  exp_bits=8  fraction_bits=24  quantization=Truncate  overflow=Wrap  en=off  latency=0  dbl_ovrd=off  pipeline=off  block_type=convert
      settings: xl_area=[0, 0, 0, 0, 0, 0, 0]
  convert_we : xbsIndex_r4/Convert  gui_display_data_type=Fixed-point  arith_type=Unsigned  n_bits=1  bin_pt=0  float_type=Single  exp_bits=8  fraction_bits=24  quantization=Truncate  overflow=Wrap  en=off  latency=0  dbl_ovrd=off  pipeline=off  block_type=convert
      settings: xl_area=[0, 0, 0, 0, 0, 0, 0]
  mc64_hb_43_noise_snap1_bram_addr : xbsIndex_r4/Gateway Out  hdl_port=on  timing_constraint=None  locs_specified=off  LOCs={'A5','B9','A9','C1','A3','G6','E9','A6','A7','A8','B8','B1','B3','D9','B5','B4','B6','C2'}  block_type=gatewayout
      settings: infoedit="Gateway out block.  Converts Xilinx fixed point inputs into ouputs of type Simulink integer, double, or fixed point.<P><P>Hardware notes:  In hardware these blocks become top level output ports or are discarded, depending on how they are configured."  xl_area=[0, 0, 0, 0, 0, 0, 0]  sginterface={'Nallatech'=>{'xdspkit'=>{'non_memory_mapped_port'=>'uprev_Shared_BRAM_addr'}},'Xilinx'=>{'jtaghwcosim'=>{'non_memory_mapped_port'=>'uprev_Shared_BRAM_addr'},'xdspkit'=>{'non_memory_mapped_port'=>'uprev_Shared_BRAM_addr'}}}
  mc64_hb_43_noise_snap1_bram_data_in : xbsIndex_r4/Gateway Out  hdl_port=on  timing_constraint=None  locs_specified=off  LOCs={'B21','B22','A22','B23','B19','C19','A20','A21','A23','B24','A24','A25','E18','D18','C18','B18'}  block_type=gatewayout
      settings: infoedit="Gateway out block.  Converts Xilinx fixed point inputs into ouputs of type Simulink integer, double, or fixed point.<P><P>Hardware notes:  In hardware these blocks become top level output ports or are discarded, depending on how they are configured."  xl_area=[0, 0, 0, 0, 0, 0, 0]  sginterface={'Nallatech'=>{'xdspkit'=>{'non_memory_mapped_port'=>'uprev_Shared_BRAM_data_in'}},'Xilinx'=>{'jtaghwcosim'=>{'non_memory_mapped_port'=>'uprev_Shared_BRAM_data_in'},'xdspkit'=>{'non_memory_mapped_port'=>'uprev_Shared_BRAM_data_in'}}}
  mc64_hb_43_noise_snap1_bram_data_out : xbsIndex_r4/Gateway In  gui_display_data_type=Fixed-point  arith_type=Unsigned  n_bits=data_width  bin_pt=data_bin_pt  preci_type=Single  exp_width=8  frac_width=24  quantization=Truncate  overflow=Wrap  period=sample_rate  dbl_ovrd=off  timing_constraint=None  locs_specified=off  LOCs={}  hdl_port=on  block_type=gatewayin
      settings: infoedit="Gateway in block.  Converts inputs of type Simulink integer, double and fixed point to  Xilinx fixed point type.<br><br>Hardware notes:  In hardware these blocks become top level input ports."  xl_area=[0, 0, 0, 0, 0, 0, 0]
  mc64_hb_43_noise_snap1_bram_we : xbsIndex_r4/Gateway Out  hdl_port=on  timing_constraint=None  locs_specified=off  LOCs={'A14'}  block_type=gatewayout
      settings: infoedit="Gateway out block.  Converts Xilinx fixed point inputs into ouputs of type Simulink integer, double, or fixed point.<P><P>Hardware notes:  In hardware these blocks become top level output ports or are discarded, depending on how they are configured."  xl_area=[0, 0, 0, 0, 0, 0, 0]
  mem : Subsystem
  munge_in : Subsystem  AncestorBlock=casper_library_flow_control/munge  mask(munge){divisions=1, div_size=32, order=[0]}
      mask prompts: divisions "Number of divisions"; div_size "Division size (bits)"; order "Division packing order"
      mask help: Splits an input bus into the specified number of divisions and then recombines them in the order specified (most significant division = 0,least = number divisions-1)
      mask init:
      | munge_init(gcb, ...
      |     'divisions', divisions, ...
      |     'div_size', div_size, ...
      |     'order', order);
      settings: AttributesFormatString=|
      | [0]
      | 32 bits
  munge_out : Subsystem  AncestorBlock=casper_library_flow_control/munge  mask(munge){divisions=1, div_size=32, order=[0]}
      mask prompts: divisions "Number of divisions"; div_size "Division size (bits)"; order "Division packing order"
      mask help: Splits an input bus into the specified number of divisions and then recombines them in the order specified (most significant division = 0,least = number divisions-1)
      mask init:
      | munge_init(gcb, ...
      |     'divisions', divisions, ...
      |     'div_size', div_size, ...
      |     'order', order);
      settings: AttributesFormatString=|
      | [0]
      | 32 bits
  data_out : Outport
  wires:
  convert_din/1 -> munge_in/1(din)
  convert_din1/1 -> mc64_hb_43_noise_snap1_bram_data_in/1
  convert_addr/1 -> mc64_hb_43_noise_snap1_bram_addr/1
  calc_add/1(out) -> convert_addr/1
  munge_out/1(dout) -> data_out/1
  munge_in/1(dout) -> convert_din1/1
  mc64_hb_43_noise_snap1_bram_we/1 -> mem/3(In3)
  mc64_hb_43_noise_snap1_bram_data_in/1 -> mem/2(In2)
  mc64_hb_43_noise_snap1_bram_addr/1 -> mem/1(In1)
  convert_we/1 -> mc64_hb_43_noise_snap1_bram_we/1
  we/1 -> convert_we/1
  addr/1 -> calc_add/1(in)
  mc64_hb_43_noise_snap1_bram_data_out/1 -> munge_out/1(din)
  data_in/1 -> convert_din/1
  mem/1(Out1) -> mc64_hb_43_noise_snap1_bram_data_out/1

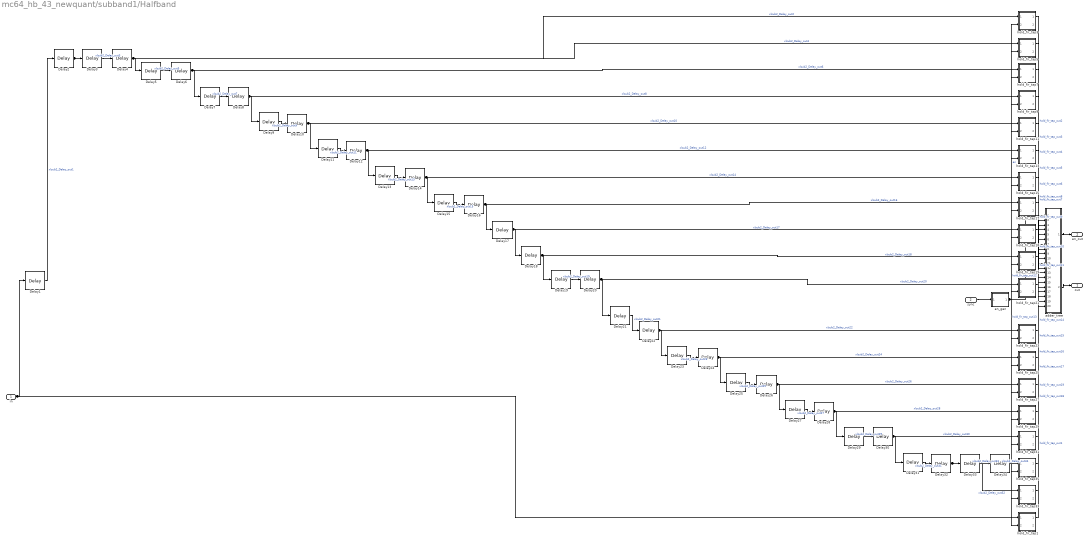
== system mc64_hb_43_newquant/subband1/Halfband ==
  in : Inport
  sync : Inport  Port=2
  Delay{1..34} (34 alike) : xbsIndex_r4/Delay  rst=off  infoeditControl=Selection of Reset will increase slice count due to use of real FFs and instead of SRLs  en=off  latency=2  dbl_ovrd=off  reg_retiming=off  block_type=delay
  adder_tree : Subsystem
      settings: AttributesFormatString=|
      | latency 10
      | hold period:2
  en_gen : Subsystem
      settings: AttributesFormatString=|
      | hold period: 2
      | explicit clk period:off , input clk period:1
  hold_fir_tap1 : Subsystem
      settings: AttributesFormatString=|
      | coefficient: 0.001155
      |  hold period: 2
      |  mult latency: 3
  hold_fir_tap11 : Subsystem
      settings: AttributesFormatString=|
      | coefficient: -0.031092
      |  hold period: 2
      |  mult latency: 3
  hold_fir_tap13 : Subsystem
      settings: AttributesFormatString=|
      | coefficient: 0.052602
      |  hold period: 2
      |  mult latency: 3
  hold_fir_tap15 : Subsystem
      settings: AttributesFormatString=|
      | coefficient: -0.099129
      |  hold period: 2
      |  mult latency: 3
  hold_fir_tap17 : Subsystem
      settings: AttributesFormatString=|
      | coefficient: 0.315926
      |  hold period: 2
      |  mult latency: 3
  hold_fir_tap18 : Subsystem
      settings: AttributesFormatString=|
      | coefficient: 0.500000
      |  hold period: 2
      |  mult latency: 3
  hold_fir_tap19 : Subsystem
      settings: AttributesFormatString=|
      | coefficient: 0.315926
      |  hold period: 2
      |  mult latency: 3
  hold_fir_tap21 : Subsystem
      settings: AttributesFormatString=|
      | coefficient: -0.099129
      |  hold period: 2
      |  mult latency: 3
  hold_fir_tap23 : Subsystem
      settings: AttributesFormatString=|
      | coefficient: 0.052602
      |  hold period: 2
      |  mult latency: 3
  hold_fir_tap25 : Subsystem
      settings: AttributesFormatString=|
      | coefficient: -0.031092
      |  hold period: 2
      |  mult latency: 3
  hold_fir_tap27 : Subsystem
      settings: AttributesFormatString=|
      | coefficient: 0.018590
      |  hold period: 2
      |  mult latency: 3
  hold_fir_tap29 : Subsystem
      settings: AttributesFormatString=|
      | coefficient: -0.010734
      |  hold period: 2
      |  mult latency: 3
  hold_fir_tap3 : Subsystem
      settings: AttributesFormatString=|
      | coefficient: -0.002747
      |  hold period: 2
      |  mult latency: 3
  hold_fir_tap31 : Subsystem
      settings: AttributesFormatString=|
      | coefficient: 0.005767
      |  hold period: 2
      |  mult latency: 3
  hold_fir_tap33 : Subsystem
      settings: AttributesFormatString=|
      | coefficient: -0.002747
      |  hold period: 2
      |  mult latency: 3
  hold_fir_tap35 : Subsystem
      settings: AttributesFormatString=|
      | coefficient: 0.001155
      |  hold period: 2
      |  mult latency: 3
  hold_fir_tap5 : Subsystem
      settings: AttributesFormatString=|
      | coefficient: 0.005767
      |  hold period: 2
      |  mult latency: 3
  hold_fir_tap7 : Subsystem
      settings: AttributesFormatString=|
      | coefficient: -0.010734
      |  hold period: 2
      |  mult latency: 3
  hold_fir_tap9 : Subsystem
      settings: AttributesFormatString=|
      | coefficient: 0.018590
      |  hold period: 2
      |  mult latency: 3
  out : Outport
  en_out : Outport  Port=2
  wires:
  in/1 -> hold_fir_tap1/1(data_in), Delay1/1
  Delay2/1 -> hold_fir_tap3/1(data_in), Delay3/1  "xlsub2_Delay_out2"
  Delay4/1 -> hold_fir_tap5/1(data_in), Delay5/1  "xlsub2_Delay_out4"
  Delay6/1 -> hold_fir_tap7/1(data_in), Delay7/1  "xlsub2_Delay_out6"
  Delay8/1 -> hold_fir_tap9/1(data_in), Delay9/1  "xlsub2_Delay_out8"
  Delay10/1 -> hold_fir_tap11/1(data_in), Delay11/1  "xlsub2_Delay_out10"
  Delay12/1 -> hold_fir_tap13/1(data_in), Delay13/1  "xlsub2_Delay_out12"
  Delay14/1 -> hold_fir_tap15/1(data_in), Delay15/1  "xlsub2_Delay_out14"
  Delay16/1 -> hold_fir_tap17/1(data_in), Delay17/1  "xlsub2_Delay_out16"
  Delay17/1 -> hold_fir_tap18/1(data_in), Delay18/1  "xlsub2_Delay_out17"
  Delay18/1 -> hold_fir_tap19/1(data_in), Delay19/1  "xlsub2_Delay_out18"
  Delay20/1 -> hold_fir_tap21/1(data_in), Delay21/1  "xlsub2_Delay_out20"
  Delay22/1 -> hold_fir_tap23/1(data_in), Delay23/1  "xlsub2_Delay_out22"
  Delay24/1 -> hold_fir_tap25/1(data_in), Delay25/1  "xlsub2_Delay_out24"
  Delay26/1 -> hold_fir_tap27/1(data_in), Delay27/1  "xlsub2_Delay_out26"
  Delay28/1 -> hold_fir_tap29/1(data_in), Delay29/1  "xlsub2_Delay_out28"
  Delay30/1 -> hold_fir_tap31/1(data_in), Delay31/1  "xlsub2_Delay_out30"
  Delay32/1 -> hold_fir_tap33/1(data_in), Delay33/1  "xlsub2_Delay_out32"
  en_gen/1(en_out) -> adder_tree/1(en_in), hold_fir_tap35/2(en_in), hold_fir_tap33/2(en_in), hold_fir_tap31/2(en_in), hold_fir_tap29/2(en_in), hold_fir_tap27/2(en_in), hold_fir_tap25/2(en_in), hold_fir_tap23/2(en_in), hold_fir_tap21/2(en_in), hold_fir_tap19/2(en_in), hold_fir_tap18/2(en_in), hold_fir_tap17/2(en_in), hold_fir_tap15/2(en_in), hold_fir_tap13/2(en_in), hold_fir_tap11/2(en_in), hold_fir_tap9/2(en_in), hold_fir_tap7/2(en_in), hold_fir_tap5/2(en_in), hold_fir_tap3/2(en_in), hold_fir_tap1/2(en_in)  "en"
  adder_tree/2(dout) -> out/1
  adder_tree/1(en_out) -> en_out/1
  hold_fir_tap35/1(mult_out) -> adder_tree/20(din19)  "hold_fir_tap_out19"
  hold_fir_tap33/1(mult_out) -> adder_tree/19(din18)  "hold_fir_tap_out18"
  hold_fir_tap31/1(mult_out) -> adder_tree/18(din17)  "hold_fir_tap_out17"
  hold_fir_tap29/1(mult_out) -> adder_tree/17(din16)  "hold_fir_tap_out16"
  hold_fir_tap27/1(mult_out) -> adder_tree/16(din15)  "hold_fir_tap_out15"
  hold_fir_tap25/1(mult_out) -> adder_tree/15(din14)  "hold_fir_tap_out14"
  hold_fir_tap23/1(mult_out) -> adder_tree/14(din13)  "hold_fir_tap_out13"
  hold_fir_tap21/1(mult_out) -> adder_tree/13(din12)  "hold_fir_tap_out12"
  hold_fir_tap19/1(mult_out) -> adder_tree/12(din11)  "hold_fir_tap_out11"
  hold_fir_tap18/1(mult_out) -> adder_tree/11(din10)  "hold_fir_tap_out10"
  hold_fir_tap17/1(mult_out) -> adder_tree/10(din9)  "hold_fir_tap_out9"
  hold_fir_tap15/1(mult_out) -> adder_tree/9(din8)  "hold_fir_tap_out8"
  hold_fir_tap13/1(mult_out) -> adder_tree/8(din7)  "hold_fir_tap_out7"
  hold_fir_tap11/1(mult_out) -> adder_tree/7(din6)  "hold_fir_tap_out6"
  hold_fir_tap9/1(mult_out) -> adder_tree/6(din5)  "hold_fir_tap_out5"
  hold_fir_tap7/1(mult_out) -> adder_tree/5(din4)  "hold_fir_tap_out4"
  hold_fir_tap5/1(mult_out) -> adder_tree/4(din3)  "hold_fir_tap_out3"
  hold_fir_tap3/1(mult_out) -> adder_tree/3(din2)  "hold_fir_tap_out2"
  hold_fir_tap1/1(mult_out) -> adder_tree/2(din1)  "hold_fir_tap_out1"
  Delay34/1 -> hold_fir_tap35/1(data_in)  "xlsub2_Delay_out34"
  Delay33/1 -> Delay34/1  "xlsub2_Delay_out33"
  Delay31/1 -> Delay32/1  "xlsub2_Delay_out31"
  Delay29/1 -> Delay30/1  "xlsub2_Delay_out29"
  Delay27/1 -> Delay28/1  "xlsub2_Delay_out27"
  Delay25/1 -> Delay26/1  "xlsub2_Delay_out25"
  Delay23/1 -> Delay24/1  "xlsub2_Delay_out23"
  Delay21/1 -> Delay22/1  "xlsub2_Delay_out21"
  Delay19/1 -> Delay20/1  "xlsub2_Delay_out19"
  Delay15/1 -> Delay16/1  "xlsub2_Delay_out15"
  Delay13/1 -> Delay14/1  "xlsub2_Delay_out13"
  Delay11/1 -> Delay12/1  "xlsub2_Delay_out11"
  Delay9/1 -> Delay10/1  "xlsub2_Delay_out9"
  Delay7/1 -> Delay8/1  "xlsub2_Delay_out7"
  Delay5/1 -> Delay6/1  "xlsub2_Delay_out5"
  Delay3/1 -> Delay4/1  "xlsub2_Delay_out3"
  Delay1/1 -> Delay2/1  "xlsub2_Delay_out1"
  sync/1 -> en_gen/1(sync_in)
